simulink model "Car_1_Jan_downsizewithbetteroutput"  (Simulink 8.1)
settings: Solver=ode5  StartTime=0.0  StopTime=inf  FixedStep=sample_time  RelTol=1e-3
InitFcn:
  | sample_time=0.005;%0.004;%0.0025;%0.02;
  | sample_time_Vicon = 0.005;
  | DeltaT = 0.02;
  | g = 9.81;
  | H0 = g%0.3165;
  | Kl = 1;
  | 
  | Q6_mass = 0.84;
  | 
  | Q6_Omega_r = 1.5; %for horizon ref
  | Q6_Zeta_r = 0.5; %for horizon ref
  | Q6_Omega_r_h = 2;%for vertical ref
  | Q6_Zeta_r_h = 2; %for vertical ref
  | 
  | 
  | Q6_Omega = 1.5; %for horizon control
  | Q6_Zeta = 0.5; %for horizon control
  | Q6_Omega_h= 2; %for vertical control
  | Q6_Zeta_h = 0.7; %for vertical control
  | 
  | 
  | Q6_acc_max = 5;%horizontal max acc
  | Q6_acc_max_h = 3;%horizontal max acc
  | 
  | omega_circle = 72*pi/180;
  | omega_h = 0.1;%Ascending speed
  | PI = pi;
  | Circle_R = 2.5;
  | MAX_Height = -2;
undefined symbols (not defined in the file or in its folder): DiscIntNeverNeededParam, fdesignblkfcn, gcbh
libraries: simulink x12, X330_Control x3
(part 2 of 2)

== stateflow chart UAV 1/Trajectory Logic/stateflowforwholesequence ==
  state Landing
    state Decsending
      en:PosDesired = Pos;
      du:PosDesired[2] = (0 - PosDesired[2])*1*DeltaT + PosDesired[2] ;
    state CutThrottle
      du:HoverThrottle = (0.01 - HoverThrottle)*2*DeltaT + HoverThrottle ;
    (default) -> Landing.Decsending
    Landing.Decsending -> Landing.CutThrottle : [Pos[2] > -0.22]
  state Airborne1
    state TakeOff
      du:HoverThrottle = (H0 - HoverThrottle)*2*DeltaT + HoverThrottle ;
    state capturing_sequence
      state normal_capturing2
        en: PosDesired[0] = car[0] ; PosDesired[1] = car[1]; PosDesired[2] = -0.5;
      state movetoLA
        en: PosDesired[2] = -1.3; PosDesired[0] = landing_area[0];PosDesired[1] = 0;
      state caputuring_test
        en: PosDesired[2] = -1.3
      state prepare_move_LA
        en: PosDesired[2] = -1.3; PosDesired[0] = 0;PosDesired[1] = 0;
      state movetoLAfinish
        en: PosDesired[2] = -1.3; PosDesired[0] = landing_area[0];PosDesired[1] = landing_area[1];
      state move_out_from_LA
        en: PosDesired[2] = -1.3; PosDesired[0] = landing_area[0];PosDesired[1] = 0;
      state CutThrottle
        du:HoverThrottle = (0.01 - HoverThrottle)*2*DeltaT + HoverThrottle ;
      state move_out_to_origin
        en: PosDesired[2] = -0.6; PosDesired[0] = 0;PosDesired[1] = 0;
      state Decsending
        du:PosDesired[2] = (-0.8 - PosDesired[2])*1*DeltaT + PosDesired[2] ;
      state normal_capturing1
        en: PosDesired[0] = carest[0] + 0.3*(car[0] - Pos[0])/abs(car[0] - Pos[0]); PosDesired[1] = carest[1] + 0.3*(car[1] - Pos[1])/(abs(car[1] - Pos[1])); PosDesired[2] = -0.5;
      (default) -> move_out_from_LA
      move_out_from_LA -> move_out_to_origin : after(5,sec)
      move_out_to_origin -> normal_capturing1 : after(5,sec)
      caputuring_test -> normal_capturing1 [order 1] : [pos[2] - car[2] <-0.6 && pos[2]<-1]
      normal_capturing1 -> caputuring_test [order 2] : [abs(Pos[0] - car[0])+abs(Pos[1] - car[1]) < 0.2]
      normal_capturing2 -> normal_capturing1 [order 1] : after(1,sec)
      normal_capturing1 -> normal_capturing2 [order 1] : after(1,sec)
      normal_capturing2 -> caputuring_test [order 2] : [abs(Pos[0] - car[0])+abs(Pos[1] - car[1]) < 0.2]
      caputuring_test -> prepare_move_LA [order 2] : [pos[2] - car[2] >-0.6 && pos[2] - car[2]<-0.4 &&pos[2]<-1.25]
      prepare_move_LA -> movetoLA : after(5,sec)
      movetoLA -> movetoLAfinish : after(5,sec)
      movetoLAfinish -> Airborne1.capturing_sequence.Decsending : [(abs(Pos[0]-PosDesired[0])+abs(Pos[1]-PosDesired[1]))<0.02]
      Airborne1.capturing_sequence.Decsending -> Airborne1.capturing_sequence.CutThrottle : [Pos[2] > -0.8]
    state Hover
      en: PosDesired[2] = -1.3;
    (default) -> TakeOff : {PosDesired[0] = landing_area[0];PosDesired[1] = landing_area[1] ; PosDesired[2] = -1.3;}
    TakeOff -> Hover : after(5,sec)
    Hover -> capturing_sequence : [RC[5] > 0]
    capturing_sequence -> Hover : [RC[5] < 0]
        | {PosDesired = Pos;}
  Landing -> Airborne1 : [RC[6] > 0.5]
  Airborne1 -> Landing : [RC[6] < -0.5]
  (default) -> Landing : {HoverThrottle=0.01;}
  data: PosDesired output double size=4; HoverThrottle output double size=1; RC input double size=8; Pos input double size=4; DeltaT parameter double size=1; H0 parameter double size=1; Kl parameter double size=1; VelCmd local double size=2 =0; line_count local int8 size=1 =0; triangle_count local int8 size=1 =0; T_line local double size=1; omega_circle parameter double size=1; PI parameter double size=1; omega_h parameter double; Circle_R parameter double size=1; MAX_Height parameter double size=1; landing_area input double size=6; car input double size=6; carest input double size=2

== matlab function UAV 1/Vertical Controller/Verticall Pos Controller/MATLAB Function ==
  data: match_flag input double; mass output double
function mass = fcn(match_flag)
%#codegen
if(match_flag == 1)
    mass = 1.12;
else
    mass = 0.84;
end
